simulink model "simulacao"  (R2018a)
settings: Solver=VariableStepAuto  StartTime=0.0  StopTime=1000  RelTol=1e-3
undefined symbols (not defined in the file): denC, deng, dengR, Kd, Ki, Kp, Kw, numC, numg, numgR
settings Model: Creator=VITOR  LastModifiedBy=VITOR

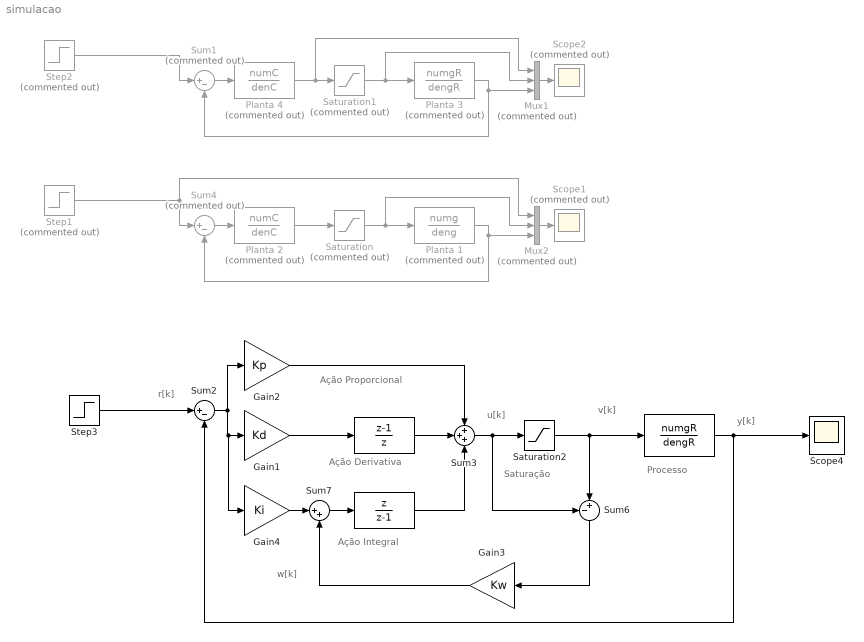
== system simulacao ==
  note: Ação Proporcional
  note: Ação Derivativa
  note: Ação Integral
  note: Processo
  note: y[k]
  note: Saturação
  note: r[k]
  note: w[k]
  note: v[k]
  note: u[k]
  " " : DiscreteTransferFcn  Numerator=numgR  Denominator=dengR  SampleTime=0.5
  " " : DiscreteTransferFcn  Numerator=[1 0]  Denominator=[1 -1]  SampleTime=0.5
  "            " : DiscreteTransferFcn  Numerator=[1 -1]  Denominator=[1 0]  SampleTime=0.5
  Gain1 : Gain  Gain=Kd
  Gain2 : Gain  Gain=Kp
  Gain3 : Gain  Gain=Kw
  Gain4 : Gain  Gain=Ki
  Mux1 : Mux  Commented=on  Inputs=3
  Mux2 : Mux  Commented=on  Inputs=3
  Planta 1 : DiscreteTransferFcn  Commented=on  Numerator=numg  Denominator=deng  SampleTime=0.5
  Planta 2 : DiscreteTransferFcn  Commented=on  Numerator=numC  Denominator=denC  SampleTime=0.5
  Planta 3 : DiscreteTransferFcn  Commented=on  Numerator=numgR  Denominator=dengR  SampleTime=0.5
  Planta 4 : DiscreteTransferFcn  Commented=on  Numerator=numC  Denominator=denC  SampleTime=0.5
  Saturation : Saturate  Commented=on  UpperLimit=10  LowerLimit=0
  Saturation1 : Saturate  Commented=on  UpperLimit=10  LowerLimit=0
  Saturation2 : Saturate  UpperLimit=10  LowerLimit=0
  Scope1 : Scope  Commented=on
  Scope2 : Scope  Commented=on
  Scope4 : Scope
  Step1 : Step  Commented=on  Time=0  After=5  SampleTime=0
  Step2 : Step  Commented=on  Time=0  After=5  SampleTime=0
  Step3 : Step  Time=0  After=7.5  SampleTime=0
  Sum1 : Sum  Commented=on  Inputs=|+-
  Sum2 : Sum  Inputs=|+-
  Sum3 : Sum  Inputs=+++
  Sum4 : Sum  Commented=on  Inputs=|+-
  Sum6 : Sum  Inputs=-+|
  Sum7 : Sum  Inputs=|++
  wires:
  Step1/1 -> Sum4/1, Mux2/1
  Planta 1/1 -> Mux2/3, Sum4/2
  Sum4/1 -> Planta 2/1
  Mux2/1 -> Scope1/1
  Saturation/1 -> Mux2/2, Planta 1/1
  Planta 2/1 -> Saturation/1
  Sum1/1 -> Planta 4/1
  Planta 3/1 -> Mux1/3, Sum1/2
  Mux1/1 -> Scope2/1
  Saturation1/1 -> Mux1/2, Planta 3/1
  Planta 4/1 -> Mux1/1, Saturation1/1
  Step2/1 -> Sum1/1
  Sum2/1 -> Gain4/1, Gain1/1, Gain2/1
  " "/1 -> Sum2/2, Scope4/1
  " "/1 -> Sum3/3
  "            "/1 -> Sum3/2
  Gain2/1 -> Sum3/1
  Gain1/1 -> "            "/1
  Sum3/1 -> Sum6/1, Saturation2/1
  Step3/1 -> Sum2/1
  Sum6/1 -> Gain3/1
  Sum7/1 -> " "/1
  Gain3/1 -> Sum7/2
  Saturation2/1 -> " "/1, Sum6/2
  Gain4/1 -> Sum7/1
